simulink model "RealesPendel"  (R2024b)
settings: Solver=VariableStepAuto  StartTime=0.0  StopTime=30  RelTol=1e-3
settings Model: Creator=Aleksandar  LastModifiedBy=Aleksandar

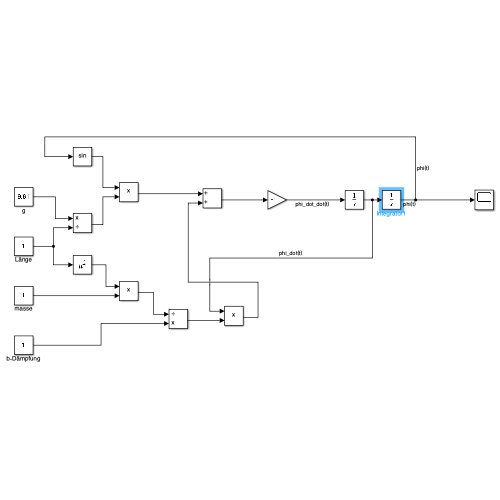
[thumbnail: Simulink's stored preview of the top-level diagram]
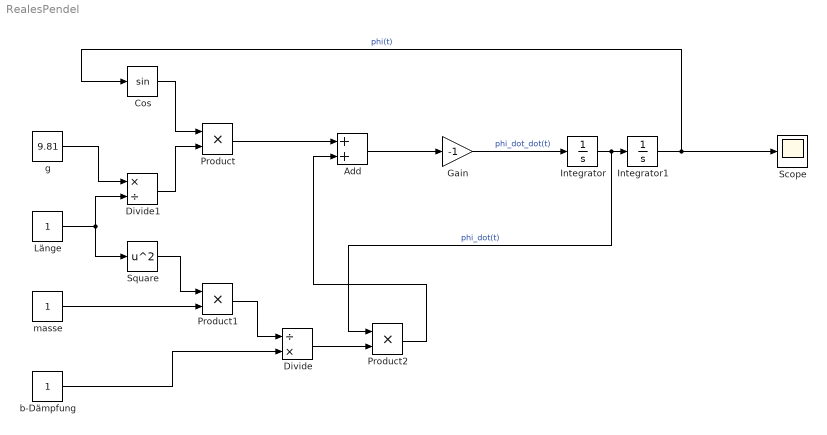
== system RealesPendel ==
  Add : Sum
  Cos : Trigonometry
  Divide : Product  Inputs=/*
  Divide1 : Product  Inputs=*/
  Gain : Gain  Gain=-1
  Integrator : Integrator
  Integrator1 : Integrator  InitialCondition=-1.309
  Länge : Constant
  Product : Product
  Product1 : Product
  Product2 : Product
  Scope : Scope
  Square : Math  Operator=square
  b-Dämpfung : Constant
  g : Constant  Value=9.81
  masse : Constant
  wires:
  g/1 -> Divide1/1
  Länge/1 -> Square/1, Divide1/2
  Integrator/1 -> Product2/1, Integrator1/1  "phi_dot(t)"
  Gain/1 -> Integrator/1  "phi_dot_dot(t)"
  Integrator1/1 -> Scope/1, Cos/1  "phi(t)"
  Divide1/1 -> Product/2
  Cos/1 -> Product/1
  Square/1 -> Product1/1
  masse/1 -> Product1/2
  Product1/1 -> Divide/1
  b-Dämpfung/1 -> Divide/2
  Divide/1 -> Product2/2
  Product/1 -> Add/1
  Product2/1 -> Add/2
  Add/1 -> Gain/1
